simulink model "MPC_regul"  (R2017a)
settings: Solver=VariableStepAuto  StartTime=0.0  StopTime=100  RelTol=1e-3
values from neighbouring files (symbols this model uses):
  P_0 = eye(8)*100    [MPC_setup.m]
  R1 = sqrtm(R)    [MPC_setup.m]
  Ts_control = 0.05    [MPC_setup.m]
  Ts_kalman = 0.01    [MPC_setup.m]
  x_0 = [0,0,0,0,0,0,0,0]    [MPC_setup.m]
settings Model: Creator=sverreknutsen  LastModifiedBy=sverreknutsen
settings SolverCC: AlgebraicLoopSolver=LineSearch

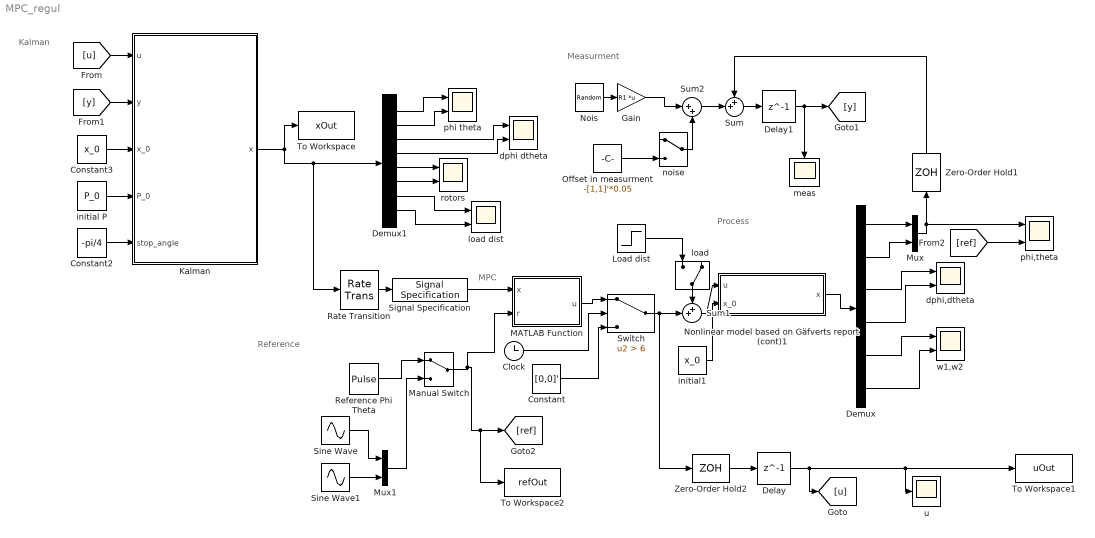
== system MPC_regul ==
  note: Process
  note: Measurment
  note: MPC
  note: Kalman
  note: Reference
  Clock : Clock
  Constant : Constant  Value=[0,0]'
  Constant2 : Constant  Value=-pi/4
  Constant3 : Constant  Value=x_0
  Delay : Delay  DelayLength=1
  Delay1 : Delay  DelayLength=1
  Demux : Demux  Outputs=6
  Demux1 : Demux  Outputs=8
  Gain : Gain  Gain=R1  Multiplication=Matrix(K*u)
  Kalman : MATLAB Function  TreatAsAtomicUnit=on
  Load dist : Step  Time=30  Before=[0,0]'  After=[1,0]'*0.2  SampleTime=0
  MATLAB Function : MATLAB Function  TreatAsAtomicUnit=on
  Manual Switch : ManualSwitch
  Mux : Mux  Inputs=2
  Mux1 : Mux  Inputs=2
  Nois : RandomNumber  Mean=[0,0]'  Variance=[1,1]'  Seed=[1,2]  SampleTime=Ts_kalman
  Nonlinear model based on Gäfverts report (cont)1 : Subsystem
  Offset in measurment : Constant  Value=-[1,1]'*0.05
  Rate Transition : RateTransition  X0=x_0  OutPortSampleTime=Ts_control
  "Reference Phi Theta " : DiscretePulseGenerator  Amplitude=[pi/7,0]'  Period=40/Ts_control  PulseWidth=20/Ts_control  SampleTime=Ts_control
  Signal Specification : SignalSpecification  Dimensions=[8 1]  SampleTime=Ts_control
  Sine Wave : Sin  Amplitude=pi/14  Bias=-pi/14  Frequency=0.5  SampleTime=Ts_control
  Sine Wave1 : Sin  Amplitude=pi/14  Bias=-pi/14  Frequency=0.5  Phase=pi/2  SampleTime=Ts_control
  Sum : Sum  Inputs=++|
  Sum1 : Sum  Inputs=++|
  Sum2 : Sum  Inputs=|++
  Switch : Switch  Criteria=u2 > Threshold  Threshold=6
  To Workspace : ToWorkspace  VariableName=xOut  SaveFormat=Timeseries  SampleTime=-1
  To Workspace1 : ToWorkspace  VariableName=uOut  SaveFormat=Timeseries  SampleTime=-1
  To Workspace2 : ToWorkspace  VariableName=refOut  SaveFormat=Timeseries  SampleTime=-1
  Zero-Order Hold1 : ZeroOrderHold  SampleTime=Ts_kalman
  Zero-Order Hold2 : ZeroOrderHold  SampleTime=Ts_kalman
  dphi dtheta : Scope  NumInputPorts=2
  dphi,dtheta : Scope  NumInputPorts=2
  "initial P " : Constant  Value=P_0
  initial1 : Constant  Value=x_0
  "load " : ManualSwitch  CurrentSetting=0
  "load dist " : Scope  NumInputPorts=2
  "meas " : Scope
  "noise " : ManualSwitch
  phi theta : Scope  NumInputPorts=2
  phi,theta : Scope  NumInputPorts=2
  "rotors " : Scope  NumInputPorts=2
  "u " : Scope
  w1,w2 : Scope  NumInputPorts=2
  wires:
  Signal Specification/1 -> MATLAB Function/1(x)
  Kalman/1(x) -> Demux1/1, Rate Transition/1, To Workspace/1
  Demux/1 -> Mux/1
  Demux/3 -> dphi,dtheta/1
  Demux/4 -> dphi,dtheta/2
  Demux/5 -> w1,w2/1
  Demux/6 -> w1,w2/2
  Demux/2 -> Mux/2
  Nonlinear model based on Gäfverts report (cont)1/1(x) -> Demux/1
  Switch/1 -> Sum1/2, Zero-Order Hold2/1
  Constant/1 -> Switch/3
  "initial P "/1 -> Kalman/4(P_0)
  Constant3/1 -> Kalman/3(x_0)
  [u] -> Kalman/1(u)
  [y] -> Kalman/2(y)
  Mux/1 -> Zero-Order Hold1/1, phi,theta/1
  Zero-Order Hold2/1 -> Delay/1
  Rate Transition/1 -> Signal Specification/1
  Delay/1 -> [u], "u "/1, To Workspace1/1
  Sum/1 -> Delay1/1
  Sum1/1 -> Nonlinear model based on Gäfverts report (cont)1/1(u)
  "load "/1 -> Sum1/1
  Load dist/1 -> "load "/1
  Clock/1 -> Switch/2
  initial1/1 -> Nonlinear model based on Gäfverts report (cont)1/2(x_0)
  MATLAB Function/1(u) -> Switch/1
  Demux1/8 -> "load dist "/2
  Demux1/7 -> "load dist "/1
  Demux1/1 -> phi theta/1
  Demux1/2 -> phi theta/2
  Demux1/3 -> dphi dtheta/1
  Demux1/4 -> dphi dtheta/2
  Delay1/1 -> [y], "meas "/1
  Nois/1 -> Gain/1
  Gain/1 -> Sum2/1
  Demux1/5 -> "rotors "/1
  Demux1/6 -> "rotors "/2
  Sum2/1 -> Sum/2
  Zero-Order Hold1/1 -> Sum/1
  Sine Wave1/1 -> Mux1/2
  Sine Wave/1 -> Mux1/1
  "Reference Phi Theta "/1 -> Manual Switch/1
  Mux1/1 -> Manual Switch/2
  "noise "/1 -> Sum2/2
  Offset in measurment/1 -> "noise "/2
  Constant2/1 -> Kalman/5(stop_angle)
  [ref] -> phi,theta/2
  Manual Switch/1 -> To Workspace2/1, [ref], MATLAB Function/2(r)

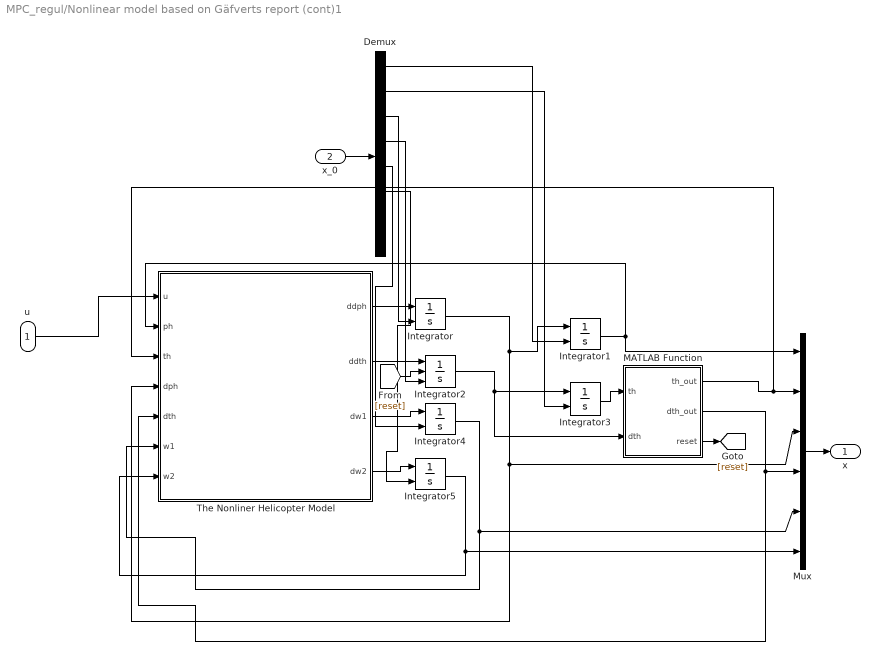
== system MPC_regul/Nonlinear model based on Gäfverts report (cont)1 ==
  u : Inport
  x_0 : Inport  Port=2
  Demux : Demux  Outputs=8
  Integrator{,1,4..5} (4 alike) : Integrator  InitialConditionSource=external
  Integrator2 : Integrator  ExternalReset=rising  InitialConditionSource=external  ShowStatePort=on
  Integrator3 : Integrator  InitialConditionSource=external  ShowStatePort=on
  MATLAB Function : MATLAB Function  TreatAsAtomicUnit=on
  Mux : Mux  Inputs=6
  The Nonliner Helicopter Model : MATLAB Function  TreatAsAtomicUnit=on
  x : Outport
  wires:
  u/1 -> The Nonliner Helicopter Model/1(u)
  The Nonliner Helicopter Model/1(ddph) -> Integrator/1
  Integrator/1 -> The Nonliner Helicopter Model/4(dph), Mux/3, Integrator1/1
  The Nonliner Helicopter Model/2(ddth) -> Integrator2/1
  The Nonliner Helicopter Model/3(dw1) -> Integrator4/1
  The Nonliner Helicopter Model/4(dw2) -> Integrator5/1
  Integrator5/1 -> The Nonliner Helicopter Model/7(w2), Mux/6
  Integrator4/1 -> The Nonliner Helicopter Model/6(w1), Mux/5
  Integrator1/1 -> Mux/1, The Nonliner Helicopter Model/2(ph)
  Integrator3/1 -> MATLAB Function/1(th)
  Mux/1 -> x/1
  x_0/1 -> Demux/1
  Integrator2/1 -> Integrator3/1, MATLAB Function/2(dth)
  MATLAB Function/1(th_out) -> The Nonliner Helicopter Model/3(th), Mux/2
  MATLAB Function/2(dth_out) -> The Nonliner Helicopter Model/5(dth), Mux/4
  MATLAB Function/3(reset) -> [reset]
  [reset] -> Integrator2/2
  Demux/1 -> Integrator1/2
  Demux/2 -> Integrator3/2
  Demux/3 -> Integrator/2
  Demux/4 -> Integrator2/3
  Demux/5 -> Integrator4/2
  Demux/6 -> Integrator5/2

== matlab function MPC_regul/MATLAB Function ==
  data: x input; u output; r input
function u = MPC(x,r)
%The MPC solver using CVXgen. 

coder.extrinsic('mycsolve'); %force simulink to accept that mycsolve will acctualy return u in a vector.
u = [0;0]; % pre-define u to be of correct type/size [u] = mycsolve(x);

% if(isempty(x)) %initialize
%     x=x_0;
%     u=mycsolve(x); %solve
% 
% else

    u=mycsolve(x,r); %solve
end

== matlab function MPC_regul/Kalman ==
  data: u input; x output; y input; x_0 input; P_0 input; stop_angle input
function x = extended_kalman(u,y,x_0,P_0,stop_angle)
persistent x_hat;
persistent P;
if(isempty(x_hat))
    x_hat=x_0;
    P=P_0;
end
coder.extrinsic('updateKalman');

[x_hat,P]=updateKalman(x_hat,u,y,P,stop_angle);
x=x_hat;

== matlab function MPC_regul/Nonlinear model based on Gäfverts report (cont)1/MATLAB Function ==
  data: th input; th_out output; dth input; dth_out output; reset output
function [th_out,dth_out,reset] = fcn(th,dth)

if(th<=-pi/4&&dth<0)
    th_out=-pi/4;
    dth_out=0;
    reset=1;
else
    th_out=th;
    dth_out=dth; 
    reset=0;
end

== matlab function MPC_regul/Nonlinear model based on Gäfverts report (cont)1/The Nonliner Helicopter Model ==
  data: u input; ddph output; ph input; th input; dph input; dth input; w1 input; w2 input; ddth output; dw1 output; dw2 output
function [ddph, ddth, dw1, dw2] = fcn(u, ph, th, dph, dth, w1, w2)
% Implementation of the non-linear integration model derived in the
% technical report "Modelling of the ETH Helicopter Laboratory Process"
% by Magnus Gäfvert, implemented by Marcus Greiff for the project course in
% FRTN01/FRTN15 2018-03-18. The notation and nomenclature vollows the
% report, however, the state vector is defined as
%
%   $x \triangleq [phi; theta; \dot{phi}; \dot{theta}; \omega_1; \omega_2]$
%
% The parameters in Gäfverts report are hard coded in the non-linear model,
% but will be made more general in future revisions.


%% Parameters
% Weights
ml = 0.280;  % [kg]
m1 = 0.3792; % [kg]
m2 = 0.1739; % [kg]
mw = 0.158;  % [kg]
m  = ml + m1 + m2 + mw; % [kg] (eq. 24)

% Distances
l1 = 0.1995; % [m]
l2 = 0.1743; % [m]
lw = 0.090;  % [m]
h  = 0.0298; % [m]
lc = (ml*(l1-l2)+m1*l1-m2*l2-mw*lw)/m; % [m] (eq. 27)

% Inertial parameters
g = 9.81; % [m/s^2]
Ja = 0;   % [] (eq. 26)
Jl = (ml/3)*((l1^3+l2^3)/(l1+l2))+m1*l1^2+m2*l2^2+mw*lw^2; % [] (eq. 25)

% Time, motor and aerodynamics constants
k1 = 1.00e-2; % [Vs/rad]
k2 = 1.39e-2; % [Vs/rad]
C1 = 2.50e-5; % [Ns^/rad^2]
C2 = 1.58e-6; % [Ns^/rad^2]
D1 = 2.90e-7; % [Nms^/rad^2]
D2 = 1.76e-7; % [Nms^/rad^2]
T1 = 1.10;    % [s]
T2 = 0.33;    % [s]


%% Pre-computation of angles and extraction of states
cth = cos(th);
sth = sin(th);
u1 = u(1);
u2 = u(2);

%%rotation stop


%% Integration model
ddph = (cth^2*Jl - 2*h*cth*sth*m*lc + h^2*sth^2*m + Ja)\...
       (2*cth*sth*dph*dth*Jl - 2*h*(sth^2-cth^2)*dph*dth*m*lc - ...
	2*h^2*sth*cth*dph*dth*m + D1*w1*abs(w1)*cth + l2*cth*C2*w2*abs(w2));
ddth = (Jl + h^2*m)\...
       (-cth*sth*dph^2*Jl - h*(-sth^2+cth^2)*dph^2*m*lc - g*cth*m*lc ...
	+ h^2*sth*cth*dph^2*m + m*g*h*sth + l1*C1*w1*abs(w1) + D2*w2*abs(w2));
dw1 = -w1/T1 + u1/(k1*T1);
dw2 = -w2/T2 + u2/(k2*T2);

if(th<=-pi/4&&dth<=0&&ddth<0)
    ddth=0;
end
